simulink model "emeregency_scenario_simulation"  (R2024b)
settings: Solver=VariableStepAuto  StartTime=0.0  StopTime=20000  RelTol=1e-3
undefined symbols (not defined in the file or in its folder): m, n
libraries: dspmathops x1
settings Model: Creator=Alize  LastModifiedBy=Alize

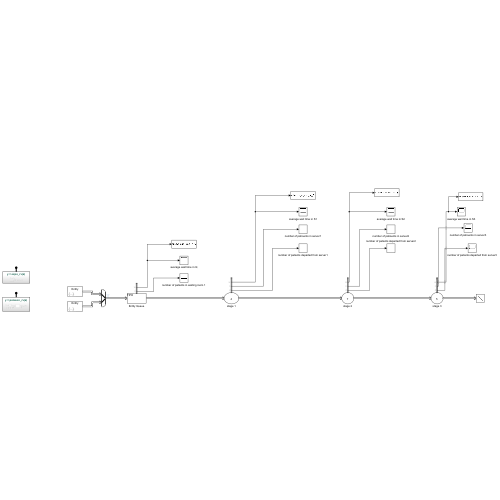
[thumbnail: Simulink's stored preview of the top-level diagram]
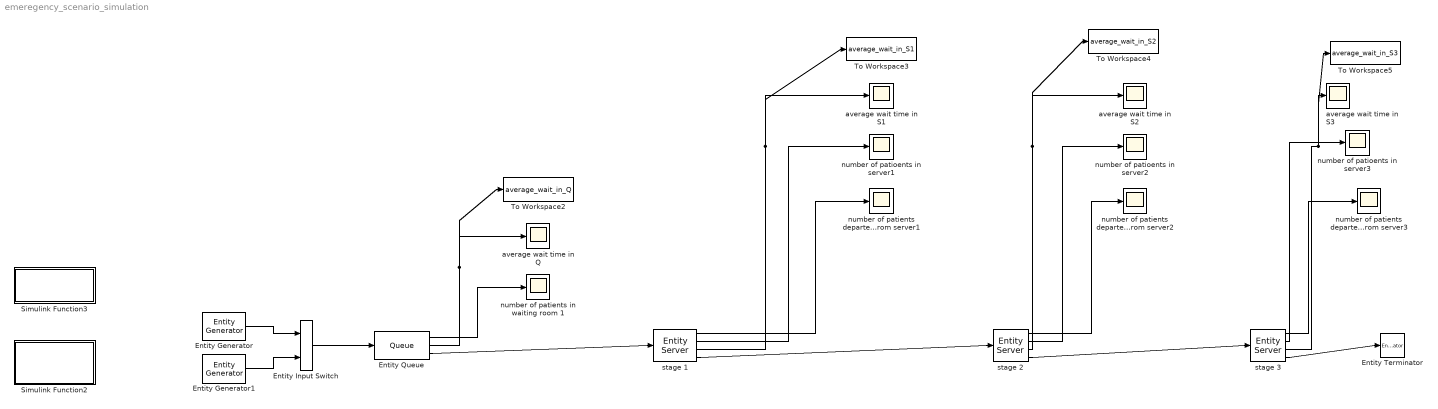
== system emeregency_scenario_simulation ==
  Entity Input Switch : EntityInputSwitch  InputPortMessageModes=m,m  OutputPortMessageModes=m
  Entity Generator : EntityGenerator  OutputPortMessageModes=m  TimeSource=MATLAB action  IntergenerationTimeAction=dt = expo_rv(1)  GenerateAction=|  AttributeName=Attribute1|Attribute2  AttributeInitialValue=1|1  EntityType=Structured  EntityTypeName=Entity
      | entity.Attribute1 = expo_rv(1);
      | entity.Attribute2 = expo_rv(1/0.5);
  Entity Generator1 : EntityGenerator  OutputPortMessageModes=m  TimeSource=MATLAB action  IntergenerationTimeAction=dt = expo_rv(2)  GenerateAction=|  AttributeName=Attribute1|Attribute2  AttributeInitialValue=1|1  EntityType=Structured  EntityTypeName=Entity
      | entity.Attribute1 = expo_rv(1/0.5);
      | entity.Attribute2 = expo_rv(1/1.5);
  Entity Queue : Queue  InputPortMessageModes=m  OutputPortMessageModes=n,n,m  Capacity=9999  NumberEntitiesInBlock=on  AverageWait=on
      settings: OutputPortMap=o1,o2,o5
  Entity Terminator : EntityTerminator  InputPortMessageModes=m
  Simulink Function2 : Subsystem  TreatAsAtomicUnit=on
  Simulink Function3 : Subsystem  TreatAsAtomicUnit=on
  To Workspace2 : ToWorkspace  VariableName=average_wait_in_Q  SaveFormat=Timeseries  SampleTime=-1
  To Workspace3 : ToWorkspace  VariableName=average_wait_in_S1  SaveFormat=Timeseries  SampleTime=-1
  To Workspace4 : ToWorkspace  VariableName=average_wait_in_S2  SaveFormat=Timeseries  SampleTime=-1
  To Workspace5 : ToWorkspace  VariableName=average_wait_in_S3  SaveFormat=Timeseries  SampleTime=-1
  average wait time in Q : Scope
  average wait time in S1 : Scope
  average wait time in S2 : Scope
  average wait time in S3 : Scope
  number of patients departed from server1 : Scope
  number of patients departed from server2 : Scope
  number of patients departed from server3 : Scope
  number of patients in waiting room 1 : Scope
  number of patioents in server1 : Scope
  number of patioents in server2 : Scope
  number of patioents in server3 : Scope
  stage 1 : EntityServer  InputPortMessageModes=m  OutputPortMessageModes=n,n,n,m  Capacity=4  ServiceTimeSource=Attribute  ServiceTimeAttributeName=Attribute1  ServiceTimeAction=dt = expo_rv(A);  NumberEntitiesDeparted=on  NumberEntitiesInBlock=on  AverageWait=on
      settings: OutputPortMap=o0,o1,o4,o9
  stage 2 : EntityServer  InputPortMessageModes=m  OutputPortMessageModes=n,n,n,m  Capacity=7  ServiceTimeSource=MATLAB action  ServiceTimeAction=dt = expo_rv(1/2);  NumberEntitiesDeparted=on  NumberEntitiesInBlock=on  AverageWait=on
      settings: OutputPortMap=o0,o1,o4,o9
  stage 3 : EntityServer  InputPortMessageModes=m  OutputPortMessageModes=n,n,n,m  ServiceTimeSource=Attribute  ServiceTimeAttributeName=Attribute2  ServiceTimeAction=dt = expo_rv(1.5);  NumberEntitiesDeparted=on  NumberEntitiesInBlock=on  AverageWait=on
      settings: OutputPortMap=o0,o1,o4,o9
  wires:
  Entity Queue/1 -> number of patients in waiting room 1/1
  stage 1/1 -> number of patients departed from server1/1
  stage 1/2 -> number of patioents in server1/1
  stage 1/4 -> stage 2/1
  stage 2/1 -> number of patients departed from server2/1
  stage 2/2 -> number of patioents in server2/1
  stage 3/1 -> number of patients departed from server3/1
  stage 3/2 -> number of patioents in server3/1
  stage 2/4 -> stage 3/1
  Entity Input Switch/1 -> Entity Queue/1
  Entity Generator1/1 -> Entity Input Switch/2
  Entity Queue/3 -> stage 1/1
  Entity Generator/1 -> Entity Input Switch/1
  stage 3/4 -> Entity Terminator/1
  stage 3/3 -> To Workspace5/1, average wait time in S3/1
  stage 2/3 -> average wait time in S2/1, To Workspace4/1
  stage 1/3 -> average wait time in S1/1, To Workspace3/1
  Entity Queue/2 -> To Workspace2/1, average wait time in Q/1

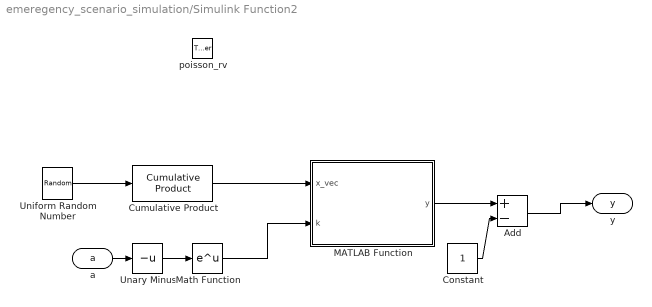
== system emeregency_scenario_simulation/Simulink Function2 ==
  poisson_rv : TriggerPort  TriggerType=function-call  IsSimulinkFunction=on  FunctionName=poisson_rv  FunctionVisibility=scoped  VariantControl=(inherit)
  Add : Sum  Inputs=+-
  Constant : Constant
  Cumulative Product : dspmathops/Cumulative Product  dim=Columns  InputProcessing=Columns as channels (frame based)  reset_popup=None  roundingMode=Floor  overflowMode=off  outputMin=[]  outputMax=[]
  MATLAB Function : MATLAB Function  TreatAsAtomicUnit=on
  Math Function : Math
  Unary Minus : UnaryMinus
  Uniform Random Number : UniformRandomNumber  Minimum=zeros(100,1)  Maximum=ones(100,1)  Seed=randi(10000,100,1)  VectorParams1D=off
  a : ArgIn  DisableCoverage=on  ArgumentName=a
  y : ArgOut  DisableCoverage=on  ArgumentName=y
  wires:
  a/1 -> Unary Minus/1
  Uniform Random Number/1 -> Cumulative Product/1
  Unary Minus/1 -> Math Function/1
  Math Function/1 -> MATLAB Function/2(k)
  Cumulative Product/1 -> MATLAB Function/1(x_vec)
  MATLAB Function/1(y) -> Add/1
  Constant/1 -> Add/2
  Add/1 -> y/1

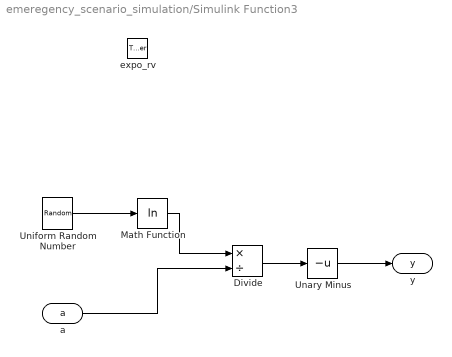
== system emeregency_scenario_simulation/Simulink Function3 ==
  expo_rv : TriggerPort  TriggerType=function-call  IsSimulinkFunction=on  FunctionName=expo_rv  FunctionVisibility=scoped  VariantControl=(inherit)
  Divide : Product  Inputs=*/
  Math Function : Math  Operator=log
  Unary Minus : UnaryMinus
  Uniform Random Number : UniformRandomNumber  Minimum=0  VectorParams1D=off
  a : ArgIn  DisableCoverage=on  ArgumentName=a
  y : ArgOut  DisableCoverage=on  ArgumentName=y
  wires:
  a/1 -> Divide/2
  Uniform Random Number/1 -> Math Function/1
  Math Function/1 -> Divide/1
  Divide/1 -> Unary Minus/1
  Unary Minus/1 -> y/1

== matlab function emeregency_scenario_simulation/Simulink Function2/MATLAB Function ==
  data: x_vec input; y output; k input
function y = first_index_lower(x_vec, k)


y = zeros(1);
y(1) = find(x_vec < k, 1, 'first');
